simulink model "Subsystem"  (R2019a)
settings: Solver=ode5  StartTime=0.0  StopTime=300  FixedStep=0.05  RelTol=1e-3
PreLoadFcn:
  | mbxruntime.callbacks.PreLoadFcn(bdroot);
PostLoadFcn:
  | mbxruntime.callbacks.PostLoadFcn(bdroot);
InitFcn:
  | mbxruntime.callbacks.InitFcn(bdroot);
StartFcn:
  | mbxruntime.callbacks.StartFcn(bdroot);
StopFcn:
  | mbxruntime.callbacks.StopFcn(bdroot);
model workspace (MAT data in the model file):
  mbox_table.root = 'ExperimentIL2209_cs'
  mbox_table.block_array(1).src = 'built-in/Subsystem'
  mbox_table.block_array(1).dest = 'Mazda_RX8_Coupe_1'
  mbox_table.block_array(1).mode = 0
  mbox_table.block_array(2).src = 'simulink/Sinks/Out1'
  mbox_table.block_array(2).dest = 'Mazda_RX8_Coupe_1/STATE_Mazda_RX8_Coupe_1_bus'
  mbox_table.block_array(2).mode = 0
  mbox_table.block_array(3).src = 'simulink/Signal Attributes/Rate Transition'
  mbox_table.block_array(3).dest = 'Mazda_RX8_Coupe_1/STATE_Mazda_RX8_Coupe_1_rc'
  mbox_table.block_array(3).mode = 0
  mbox_table.block_array(4).src = 'built-in/S-Function'
  mbox_table.block_array(4).dest = 'Mazda_RX8_Coupe_1/SpeedProfile'
  mbox_table.block_array(4).mode = 0
  mbox_table.block_array(5).src = 'built-in/S-Function'
  mbox_table.block_array(5).dest = 'Mazda_RX8_Coupe_1/Path'
  mbox_table.block_array(5).mode = 0
  mbox_table.block_array(6).src = 'simulink/Sources/In1'
  mbox_table.block_array(6).dest = 'Mazda_RX8_Coupe_1/SELF_Mazda_RX8_Coupe_1'
  mbox_table.block_array(6).mode = 0
  mbox_table.block_array(7).src = 'PreScanSimulinkLibrary/DemuxSELF'
  mbox_table.block_array(7).dest = 'Mazda_RX8_Coupe_1/SELF_Demux'
  mbox_table.block_array(7).mode = 0
  mbox_table.block_array(8).src = 'simulink/Sources/In1'
  mbox_table.block_array(8).dest = 'Mazda_RX8_Coupe_1/AIR_1'
  mbox_table.block_array(8).mode = 0
  mbox_table.block_array(9).src = 'PreScanSimulinkLibrary/DemuxAIR'
  mbox_table.block_array(9).dest = 'Mazda_RX8_Coupe_1/AIR_1_Demux'
  mbox_table.block_array(9).mode = 0
  mbox_table.block_array(10).src = 'simulink/Sources/In1'
  mbox_table.block_array(10).dest = 'Mazda_RX8_Coupe_1/CameraSensor_1'
  mbox_table.block_array(10).mode = 0
  mbox_table.block_array(11).src = 'PreScanSimulinkLibrary/Camera_Color_Demux'
  mbox_table.block_array(11).dest = 'Mazda_RX8_Coupe_1/CameraSensor_1_CM_Demux'
  mbox_table.block_array(11).mode = 0
  mbox_table.block_array(12).src = 'PreScanSimulinkLibrary/CameraSensor_Color_Display'
  mbox_table.block_array(12).dest = 'Mazda_RX8_Coupe_1/CameraSensor_1_CM_Display'
  mbox_table.block_array(12).mode = 0
  mbox_table.block_array(13).src = 'built-in/Subsystem'
  mbox_table.block_array(13).dest = 'STATE_Mazda_RX8_Coupe_1_bus'
  mbox_table.block_array(13).mode = 0
  mbox_table.block_array(14).src = 'built-in/S-Function'
  mbox_table.block_array(14).dest = 'STATE_Mazda_RX8_Coupe_1_bus/Actuator'
  mbox_table.block_array(14).mode = 0
  mbox_table.block_array(15).src = 'simulink/Sources/In1'
  mbox_table.block_array(15).dest = 'STATE_Mazda_RX8_Coupe_1_bus/STATE_Mazda_RX8_Coupe_1_bus'
  mbox_table.block_array(15).mode = 0
  mbox_table.block_array(16).src = 'built-in/Subsystem'
  mbox_table.block_array(16).dest = 'SELF_Mazda_RX8_Coupe_1'
  mbox_table.block_array(16).mode = 0
  mbox_table.block_array(17).src = 'built-in/S-Function'
  mbox_table.block_array(17).dest = 'SELF_Mazda_RX8_Coupe_1/Sensor'
  mbox_table.block_array(17).mode = 0
  mbox_table.block_array(18).src = 'simulink/Sinks/Out1'
  mbox_table.block_array(18).dest = 'SELF_Mazda_RX8_Coupe_1/SELF_Mazda_RX8_Coupe_1'
  mbox_table.block_array(18).mode = 0
  mbox_table.block_array(19).src = 'built-in/Subsystem'
  mbox_table.block_array(19).dest = 'AIR_1'
  mbox_table.block_array(19).mode = 0
  mbox_table.block_array(20).src = 'built-in/S-Function'
  mbox_table.block_array(20).dest = 'AIR_1/Sensor'
  mbox_table.block_array(20).mode = 0
  mbox_table.block_array(21).src = 'simulink/Sinks/Out1'
  mbox_table.block_array(21).dest = 'AIR_1/AIR_1'
  mbox_table.block_array(21).mode = 0
  mbox_table.block_array(22).src = 'built-in/Subsystem'
  mbox_table.block_array(22).dest = 'CameraSensor_1'
  mbox_table.block_array(22).mode = 0
  mbox_table.block_array(23).src = 'built-in/S-Function'
  mbox_table.block_array(23).dest = 'CameraSensor_1/Sensor'
  mbox_table.block_array(23).mode = 0
  mbox_table.block_array(24).src = 'simulink/Sinks/Out1'
  mbox_table.block_array(24).dest = 'CameraSensor_1/CameraSensor_1'
  mbox_table.block_array(24).mode = 0
  mbox_table.block_array(25).src = 'SimCoreLibrary/PreScanController'
  mbox_table.block_array(25).dest = 'Controller'
  mbox_table.block_array(25).mode = 0
  mbox_table.block_array(26).src = 'SimCoreLibrary/PreScanSynchronizer'
  mbox_table.block_array(26).dest = 'Synchronizer'
  mbox_table.block_array(26).mode = 0
  mbox_table.block_array(27).src = 'SimCoreLibrary/PreScanTerminator'
  mbox_table.block_array(27).dest = 'PreScanTerminator'
  mbox_table.block_array(27).mode = 0
  mbox_table.block_array(28).src = 'SimCoreLibrary/PreScanOpenScenarioEngine'
  mbox_table.block_array(28).dest = 'ScenarioEngine'
  mbox_table.block_array(28).mode = 0
  mbox_table.block_array(29).src = 'PreScanSimulinkLibrary/Regenerate'
  mbox_table.block_array(29).dest = 'Regenerate'
  mbox_table.block_array(29).mode = 0
  mbox_table.block_array(30).src = 'PreScanSimulinkLibrary/Simulink Mode'
  mbox_table.block_array(30).dest = 'Simulink Mode'
  mbox_table.block_array(30).mode = 0
  mbox_table.block_array(31).src = 'PreScanSimulinkLibrary/Open Useful Blocks'
  mbox_table.block_array(31).dest = 'Open Useful Blocks'
  mbox_table.block_array(31).mode = 0
  mbox_table.block_array(32).src = 'built-in/Note'
  mbox_table.block_array(32).dest = '2020.3.0'
  mbox_table.block_array(32).mode = 0
  mbox_table.block_array(33).src = 'built-in/Note'
  mbox_table.block_array(33).dest = 'Version:                  '
  mbox_table.block_array(33).mode = 0
  mbox_table.block_array(34).src = 'built-in/Note'
  mbox_table.block_array(34).dest = 'Author(s):                '
  mbox_table.block_array(34).mode = 0
  mbox_table.block_array(35).src = 'built-in/Note'
  mbox_table.block_array(35).dest = 'N.A.'
  mbox_table.block_array(35).mode = 0
  mbox_table.block_array(36).src = 'built-in/Note'
  mbox_table.block_array(36).dest = 'Descriptive text:      '
  mbox_table.block_array(36).mode = 0
  mbox_table.block_array(37).src = 'built-in/Note'
  mbox_table.block_array(37).dest = 'N.A.'
  mbox_table.block_array(37).mode = 0
  mbox_table.block_array(38).src = 'built-in/Note'
  mbox_table.block_array(38).dest = '======
    | Num ID
    | ======
    | 4'
  mbox_table.block_array(38).mode = 0
  mbox_table.block_array(39).src = 'built-in/Note'
  mbox_table.block_array(39).dest = '=============
    | OBU-Beacon ID
    | =============
    | '
  mbox_table.block_array(39).mode = 0
  mbox_table.block_array(40).src = 'built-in/Note'
  mbox_table.block_array(40).dest = '=======
    | Type ID
    | =======
    | 1'
  mbox_table.block_array(40).mode = 0
  mbox_table.block_array(41).src = 'built-in/Note'
  mbox_table.block_array(41).dest = '========
    | Type Tag
    | ========
    | Car'
  mbox_table.block_array(41).mode = 0
  mbox_table.block_array(42).src = 'built-in/Note'
  mbox_table.block_array(42).dest = '==
    | SD
    | ==
    | Y'
  mbox_table.block_array(42).mode = 0
  mbox_table.block_array(43).src = 'built-in/Note'
  mbox_table.block_array(43).dest = '==
    | CD
    | ==
    | N'
  mbox_table.block_array(43).mode = 0
  mbox_table.block_array(44).src = 'built-in/Note'
  mbox_table.block_array(44).dest = '=============
    | Name
    | =============
    | Mazda_RX8_Coupe_1'
  mbox_table.block_array(44).mode = 0
  mbox_table.block_array(45).src = 'built-in/Terminator'
  mbox_table.block_array(45).dest = 'Mazda_RX8_Coupe_1/Terminator_1'
  mbox_table.block_array(45).mode = 1
  mbox_table.block_array(46).src = 'built-in/Terminator'
  mbox_table.block_array(46).dest = 'Mazda_RX8_Coupe_1/Terminator_2'
  mbox_table.block_array(46).mode = 1
  mbox_table.block_array(47).src = 'built-in/Terminator'
  mbox_table.block_array(47).dest = 'Mazda_RX8_Coupe_1/Terminator_3'
  mbox_table.block_array(47).mode = 1
  mbox_table.block_array(48).src = 'built-in/Terminator'
  mbox_table.block_array(48).dest = 'Mazda_RX8_Coupe_1/Terminator_4'
  mbox_table.block_array(48).mode = 1
  mbox_table.block_array(49).src = 'built-in/Terminator'
  mbox_table.block_array(49).dest = 'Mazda_RX8_Coupe_1/Terminator_5'
  mbox_table.block_array(49).mode = 1
  mbox_table.block_array(50).src = 'built-in/Terminator'
  mbox_table.block_array(50).dest = 'Mazda_RX8_Coupe_1/Terminator_6'
  mbox_table.block_array(50).mode = 1
  mbox_table.block_array(51).src = 'built-in/Terminator'
  mbox_table.block_array(51).dest = 'Mazda_RX8_Coupe_1/Terminator_7'
  mbox_table.block_array(51).mode = 1
  mbox_table.block_array(52).src = 'built-in/Terminator'
  mbox_table.block_array(52).dest = 'Mazda_RX8_Coupe_1/Terminator_8'
  mbox_table.block_array(52).mode = 1
  mbox_table.block_array(53).src = 'built-in/Terminator'
  mbox_table.block_array(53).dest = 'Mazda_RX8_Coupe_1/Terminator_9'
  mbox_table.block_array(53).mode = 1
  mbox_table.block_array(54).src = 'built-in/Terminator'
  mbox_table.block_array(54).dest = 'Mazda_RX8_Coupe_1/Terminator_10'
  mbox_table.block_array(54).mode = 1
  mbox_table.block_array(55).src = 'built-in/Terminator'
  mbox_table.block_array(55).dest = 'Mazda_RX8_Coupe_1/Terminator_11'
  mbox_table.block_array(55).mode = 1
  mbox_table.block_array(56).src = 'built-in/Terminator'
  mbox_table.block_array(56).dest = 'Mazda_RX8_Coupe_1/Terminator_12'
  mbox_table.block_array(56).mode = 1
  mbox_table.block_array(57).src = 'built-in/Terminator'
  mbox_table.block_array(57).dest = 'Mazda_RX8_Coupe_1/Terminator_13'
  mbox_table.block_array(57).mode = 1
  mbox_table.block_array(58).src = 'built-in/Terminator'
  mbox_table.block_array(58).dest = 'Mazda_RX8_Coupe_1/Terminator_14'
  mbox_table.block_array(58).mode = 1
  mbox_table.block_array(59).src = 'built-in/Terminator'
  mbox_table.block_array(59).dest = 'Mazda_RX8_Coupe_1/Terminator_15'
  mbox_table.block_array(59).mode = 1
  mbox_table.block_array(60).src = 'built-in/Terminator'
  mbox_table.block_array(60).dest = 'Mazda_RX8_Coupe_1/Terminator_16'
  mbox_table.block_array(60).mode = 1
  mbox_table.block_array(61).src = 'built-in/Terminator'
  mbox_table.block_array(61).dest = 'Mazda_RX8_Coupe_1/Terminator_17'
  mbox_table.block_array(61).mode = 1
  mbox_table.block_array(62).src = 'built-in/Terminator'
  mbox_table.block_array(62).dest = 'Mazda_RX8_Coupe_1/Terminator_18'
  mbox_table.block_array(62).mode = 1
  mbox_table.block_array(63).src = 'built-in/Terminator'
  mbox_table.block_array(63).dest = 'Mazda_RX8_Coupe_1/Terminator_19'
  mbox_table.block_array(63).mode = 1
  mbox_table.block_array(64).src = 'built-in/Terminator'
  mbox_table.block_array(64).dest = 'Mazda_RX8_Coupe_1/Terminator_20'
  mbox_table.block_array(64).mode = 1
  mbox_table.line_array(1).sys = 'Mazda_RX8_Coupe_1'
  mbox_table.line_array(1).line_id = 'L1'
  mbox_table.line_array(1).iport = 'STATE_Mazda_RX8_Coupe_1_bus/1'
  mbox_table.line_array(1).oport = 'STATE_Mazda_RX8_Coupe_1_rc/1'
  mbox_table.line_array(1).mode = 0
  mbox_table.line_array(2).sys = 'Mazda_RX8_Coupe_1'
  mbox_table.line_array(2).line_id = 'L2'
  mbox_table.line_array(2).iport = 'Path/1'
  mbox_table.line_array(2).oport = 'SpeedProfile/1'
  mbox_table.line_array(2).mode = 0
  mbox_table.line_array(3).sys = 'Mazda_RX8_Coupe_1'
  mbox_table.line_array(3).line_id = 'L3'
  mbox_table.line_array(3).iport = 'STATE_Mazda_RX8_Coupe_1_rc/1'
  mbox_table.line_array(3).oport = 'Path/1'
  mbox_table.line_array(3).mode = 0
  mbox_table.line_array(4).sys = 'Mazda_RX8_Coupe_1'
  mbox_table.line_array(4).line_id = 'L4'
  mbox_table.line_array(4).iport = 'SELF_Demux/1'
  mbox_table.line_array(4).oport = 'SELF_Mazda_RX8_Coupe_1/1'
  mbox_table.line_array(4).mode = 0
  mbox_table.line_array(5).sys = 'Mazda_RX8_Coupe_1'
  mbox_table.line_array(5).line_id = 'L5'
  mbox_table.line_array(5).iport = 'AIR_1_Demux/1'
  mbox_table.line_array(5).oport = 'AIR_1/1'
  mbox_table.line_array(5).mode = 0
  mbox_table.line_array(6).sys = 'Mazda_RX8_Coupe_1'
  mbox_table.line_array(6).line_id = 'L6'
  mbox_table.line_array(6).iport = 'CameraSensor_1_CM_Demux/1'
  mbox_table.line_array(6).oport = 'CameraSensor_1/1'
  mbox_table.line_array(6).mode = 0
  mbox_table.line_array(7).sys = 'Mazda_RX8_Coupe_1'
  mbox_table.line_array(7).line_id = 'L7'
  mbox_table.line_array(7).iport = 'CameraSensor_1_CM_Display/1'
  mbox_table.line_array(7).oport = 'CameraSensor_1_CM_Demux/1'
  mbox_table.line_array(7).mode = 0
  mbox_table.line_array(8).sys = 'Mazda_RX8_Coupe_1'
  mbox_table.line_array(8).line_id = 'L8'
  mbox_table.line_array(8).iport = 'CameraSensor_1_CM_Display/2'
  mbox_table.line_array(8).oport = 'CameraSensor_1_CM_Demux/2'
  mbox_table.line_array(8).mode = 0
  mbox_table.line_array(9).sys = 'Mazda_RX8_Coupe_1'
  mbox_table.line_array(9).line_id = 'L9'
  mbox_table.line_array(9).iport = 'CameraSensor_1_CM_Display/3'
  mbox_table.line_array(9).oport = 'CameraSensor_1_CM_Demux/3'
  mbox_table.line_array(9).mode = 0
  mbox_table.line_array(10).sys = 'STATE_Mazda_RX8_Coupe_1_bus'
  mbox_table.line_array(10).line_id = 'L10'
  mbox_table.line_array(10).iport = 'Actuator/1'
  mbox_table.line_array(10).oport = 'STATE_Mazda_RX8_Coupe_1_bus/1'
  mbox_table.line_array(10).mode = 0
  mbox_table.line_array(11).sys = ''
  mbox_table.line_array(11).line_id = 'L11'
  mbox_table.line_array(11).iport = 'STATE_Mazda_RX8_Coupe_1_bus/1'
  mbox_table.line_array(11).oport = 'Mazda_RX8_Coupe_1/1'
  mbox_table.line_array(11).mode = 0
  mbox_table.line_array(12).sys = 'SELF_Mazda_RX8_Coupe_1'
  mbox_table.line_array(12).line_id = 'L12'
  mbox_table.line_array(12).iport = 'SELF_Mazda_RX8_Coupe_1/1'
  mbox_table.line_array(12).oport = 'Sensor/1'
  mbox_table.line_array(12).mode = 0
  mbox_table.line_array(13).sys = ''
  mbox_table.line_array(13).line_id = 'L13'
  mbox_table.line_array(13).iport = 'Mazda_RX8_Coupe_1/1'
  mbox_table.line_array(13).oport = 'SELF_Mazda_RX8_Coupe_1/1'
  mbox_table.line_array(13).mode = 0
  mbox_table.line_array(14).sys = 'AIR_1'
  mbox_table.line_array(14).line_id = 'L14'
  mbox_table.line_array(14).iport = 'AIR_1/1'
  mbox_table.line_array(14).oport = 'Sensor/1'
  mbox_table.line_array(14).mode = 0
  mbox_table.line_array(15).sys = ''
  mbox_table.line_array(15).line_id = 'L15'
  mbox_table.line_array(15).iport = 'Mazda_RX8_Coupe_1/2'
  mbox_table.line_array(15).oport = 'AIR_1/1'
  mbox_table.line_array(15).mode = 0
  mbox_table.line_array(16).sys = 'CameraSensor_1'
  mbox_table.line_array(16).line_id = 'L16'
  mbox_table.line_array(16).iport = 'CameraSensor_1/1'
  mbox_table.line_array(16).oport = 'Sensor/1'
  mbox_table.line_array(16).mode = 0
  mbox_table.line_array(17).sys = ''
  mbox_table.line_array(17).line_id = 'L17'
  mbox_table.line_array(17).iport = 'Mazda_RX8_Coupe_1/3'
  mbox_table.line_array(17).oport = 'CameraSensor_1/1'
  mbox_table.line_array(17).mode = 0
  mbox_table.line_array(18).sys = 'Mazda_RX8_Coupe_1'
  mbox_table.line_array(18).line_id = 'l1'
  mbox_table.line_array(18).iport = 'Terminator_1/1'
  mbox_table.line_array(18).oport = 'AIR_1_Demux/1'
  mbox_table.line_array(18).mode = 1
  mbox_table.line_array(19).sys = 'Mazda_RX8_Coupe_1'
  mbox_table.line_array(19).line_id = 'l2'
  mbox_table.line_array(19).iport = 'Terminator_2/1'
  mbox_table.line_array(19).oport = 'AIR_1_Demux/2'
  mbox_table.line_array(19).mode = 1
  mbox_table.line_array(20).sys = 'Mazda_RX8_Coupe_1'
  mbox_table.line_array(20).line_id = 'l3'
  mbox_table.line_array(20).iport = 'Terminator_3/1'
  mbox_table.line_array(20).oport = 'AIR_1_Demux/3'
  mbox_table.line_array(20).mode = 1
  mbox_table.line_array(21).sys = 'Mazda_RX8_Coupe_1'
  mbox_table.line_array(21).line_id = 'l4'
  mbox_table.line_array(21).iport = 'Terminator_4/1'
  mbox_table.line_array(21).oport = 'AIR_1_Demux/4'
  mbox_table.line_array(21).mode = 1
  mbox_table.line_array(22).sys = 'Mazda_RX8_Coupe_1'
  mbox_table.line_array(22).line_id = 'l5'
  mbox_table.line_array(22).iport = 'Terminator_5/1'
  mbox_table.line_array(22).oport = 'AIR_1_Demux/5'
  mbox_table.line_array(22).mode = 1
  mbox_table.line_array(23).sys = 'Mazda_RX8_Coupe_1'
  mbox_table.line_array(23).line_id = 'l6'
  mbox_table.line_array(23).iport = 'Terminator_6/1'
  mbox_table.line_array(23).oport = 'AIR_1_Demux/6'
  mbox_table.line_array(23).mode = 1
  mbox_table.line_array(24).sys = 'Mazda_RX8_Coupe_1'
  mbox_table.line_array(24).line_id = 'l7'
  mbox_table.line_array(24).iport = 'Terminator_7/1'
  mbox_table.line_array(24).oport = 'AIR_1_Demux/7'
  mbox_table.line_array(24).mode = 1
  mbox_table.line_array(25).sys = 'Mazda_RX8_Coupe_1'
  mbox_table.line_array(25).line_id = 'l8'
  mbox_table.line_array(25).iport = 'Terminator_8/1'
  mbox_table.line_array(25).oport = 'SELF_Demux/1'
  mbox_table.line_array(25).mode = 1
  mbox_table.line_array(26).sys = 'Mazda_RX8_Coupe_1'
  mbox_table.line_array(26).line_id = 'l9'
  mbox_table.line_array(26).iport = 'Terminator_9/1'
  mbox_table.line_array(26).oport = 'SELF_Demux/2'
  mbox_table.line_array(26).mode = 1
  mbox_table.line_array(27).sys = 'Mazda_RX8_Coupe_1'
  mbox_table.line_array(27).line_id = 'l10'
  mbox_table.line_array(27).iport = 'Terminator_10/1'
  mbox_table.line_array(27).oport = 'SELF_Demux/3'
  mbox_table.line_array(27).mode = 1
  mbox_table.line_array(28).sys = 'Mazda_RX8_Coupe_1'
  mbox_table.line_array(28).line_id = 'l11'
  mbox_table.line_array(28).iport = 'Terminator_11/1'
  mbox_table.line_array(28).oport = 'SELF_Demux/4'
  mbox_table.line_array(28).mode = 1
  mbox_table.line_array(29).sys = 'Mazda_RX8_Coupe_1'
  mbox_table.line_array(29).line_id = 'l12'
  mbox_table.line_array(29).iport = 'Terminator_12/1'
  mbox_table.line_array(29).oport = 'SELF_Demux/5'
  mbox_table.line_array(29).mode = 1
  mbox_table.line_array(30).sys = 'Mazda_RX8_Coupe_1'
  mbox_table.line_array(30).line_id = 'l13'
  mbox_table.line_array(30).iport = 'Terminator_13/1'
  mbox_table.line_array(30).oport = 'SELF_Demux/6'
  mbox_table.line_array(30).mode = 1
  mbox_table.line_array(31).sys = 'Mazda_RX8_Coupe_1'
  mbox_table.line_array(31).line_id = 'l14'
  mbox_table.line_array(31).iport = 'Terminator_14/1'
  mbox_table.line_array(31).oport = 'SELF_Demux/7'
  mbox_table.line_array(31).mode = 1
  mbox_table.line_array(32).sys = 'Mazda_RX8_Coupe_1'
  mbox_table.line_array(32).line_id = 'l15'
  mbox_table.line_array(32).iport = 'Terminator_15/1'
  mbox_table.line_array(32).oport = 'SELF_Demux/8'
  mbox_table.line_array(32).mode = 1
  mbox_table.line_array(33).sys = 'Mazda_RX8_Coupe_1'
  mbox_table.line_array(33).line_id = 'l16'
  mbox_table.line_array(33).iport = 'Terminator_16/1'
  mbox_table.line_array(33).oport = 'SELF_Demux/9'
  mbox_table.line_array(33).mode = 1
  mbox_table.line_array(34).sys = 'Mazda_RX8_Coupe_1'
  mbox_table.line_array(34).line_id = 'l17'
  mbox_table.line_array(34).iport = 'Terminator_17/1'
  mbox_table.line_array(34).oport = 'SELF_Demux/10'
  mbox_table.line_array(34).mode = 1
  mbox_table.line_array(35).sys = 'Mazda_RX8_Coupe_1'
  mbox_table.line_array(35).line_id = 'l18'
  mbox_table.line_array(35).iport = 'Terminator_18/1'
  mbox_table.line_array(35).oport = 'SELF_Demux/11'
  mbox_table.line_array(35).mode = 1
  mbox_table.line_array(36).sys = 'Mazda_RX8_Coupe_1'
  mbox_table.line_array(36).line_id = 'l19'
  mbox_table.line_array(36).iport = 'Terminator_19/1'
  mbox_table.line_array(36).oport = 'SELF_Demux/12'
  mbox_table.line_array(36).mode = 1
  mbox_table.line_array(37).sys = 'Mazda_RX8_Coupe_1'
  mbox_table.line_array(37).line_id = 'l20'
  mbox_table.line_array(37).iport = 'Terminator_20/1'
  mbox_table.line_array(37).oport = 'SELF_Demux/13'
  mbox_table.line_array(37).mode = 1
  mbox_table.next_linenr = 18
  mbox_table.next_termlinenr = 21
  model_closed = 0
  sim_status = 0
libraries: robotlib x2
settings Model: Creator=PRESCAN  LastModifiedBy=adeye
settings DataIOCC: LimitDataPoints=on  SaveFormat=Array  SignalLoggingSaveFormat=ModelDataLogs  SaveOutput=off  SaveTime=off  ReturnWorkspaceOutputs=off
settings OptimizationCC: EnhancedBackFolding=on  PassReuseOutputArgsAs=Individual arguments  ExpressionDepthLimit=2147483647  InitFltsAndDblsToZero=on  MaxStackSize=64  OptimizeBlockOrder=speed  DifferentSizesBufferReuse=on  OptimizationCustomize=off
settings DebuggingCC: SaveWithParameterizedLinksMsg=none  UnderspecifiedInitializationDetection=Classic  MergeDetectMultiDrivingBlocksExec=none  SignalResolutionControl=TryResolveAllWithWarning  MultiTaskDSMMsg=warning  MultiTaskCondExecSysMsg=none  ParameterTunabilityLossMsg=error  FcnCallInpInsideContextMsg=warning  StateNameClashWarn=warning  SFUnexpectedBacktrackingDiag=warning  SFNoUnconditionalDefaultTransitionDiag=warning  SFExecutionAtInitializationDiag=none  ArithmeticOperatorsInVariantConditions=warning
settings HardwareCC: ProdBitPerPointer=32  ProdBitPerSizeT=32  ProdBitPerPtrDiffT=32  ProdLargestAtomicFloat=None  ProdIntDivRoundTo=Undefined  ProdEndianess=Unspecified  ProdWordSize=32  ProdHWDeviceType=Generic->Unspecified (assume 32-bit Generic)  UseEmbeddedCoderFeatures=off
settings ModelReferenceCC: UpdateModelReferenceTargets=IfOutOfDate  PropagateSignalLabelsOutOfModel=off
settings SFSimCC: SimUseLocalCustomCode=off  SimParseCustomCode=off  MATLABDynamicMemAlloc=off
settings RTWCC: SystemTargetFile=ert.tlc  HardwareBoard=Robot Operating System (ROS)  TLCOptions="-aInlineSetEventsForThisBaseRateFcn=TLC_FALSE -aSuppressMultiTaskScheduler=TLC_FALSE  -aRateBasedStepFcn=0"  TemplateMakefile=ert_default_tmf  GenerateReport=on  RTWUseLocalCustomCode=off  Toolchain=Catkin  IncludeHyperlinkInReport=on  LaunchReport=on  TargetLang=C++  GenerateTraceInfo=on  GenerateTraceReport=on  GenerateTraceReportSl=on  GenerateTraceReportSf=on  GenerateTraceReportEml=on
settings CodeAppCC: ForceParamTrailComments=on  IgnoreCustomStorageClasses=off  OperatorAnnotations=on  SimulinkDataObjDesc=on  SFDataObjDesc=on  InsertBlockDesc=on
settings ERTTargetCC: SupportNonInlinedSFcns=on
settings ConfigComp: CovMetricSettings=dw  CovHtmlReporting=on  CovSaveCumulativeToWorkspaceVar=on  CovSaveSingleToWorkspaceVar=on  CovExternalEMLEnable=off  CovSFcnEnable=off

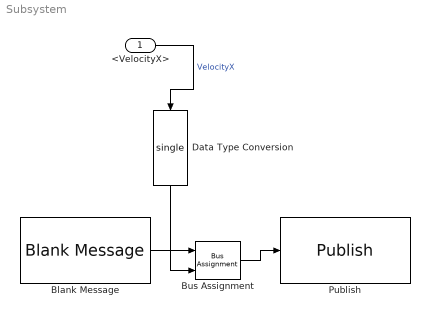
== system Subsystem ==
  <VelocityX> : Inport  OutDataTypeStr=double  PortDimensions=1  SampleTime=[0.050000000000000003,0]
  Blank Message : robotlib/Blank Message  messageClass=Message  entityType=std_msgs/Float32  messageType=std_msgs/Float32  SampleTime=inf
      settings: SourceProductBaseCode=RO
  Bus Assignment : BusAssignment  AssignedSignals=Data
  Data Type Conversion : DataTypeConversion  OutDataTypeStr=single
  Publish : robotlib/Publish  topicSource=Specify your own  topic=/velocity_x  messageType=std_msgs/Float32  messageQueueLength=1
      settings: SourceProductBaseCode=RO
  wires:
  Bus Assignment/1 -> Publish/1
  Blank Message/1 -> Bus Assignment/1
  <VelocityX>/1 -> Data Type Conversion/1  "VelocityX"
  Data Type Conversion/1 -> Bus Assignment/2
